simulink model "sys_dae"  (R2021a)
settings: Solver=VariableStepAuto  StartTime=0.0  StopTime=10.0  RelTol=1e-3
settings Model: Creator=Suman  LastModifiedBy=Suman

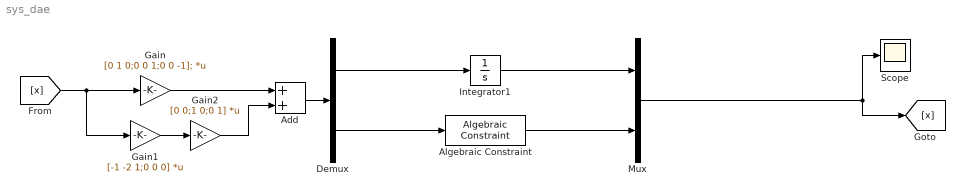
== system sys_dae ==
  Add : Sum
  Algebraic Constraint : AlgebraicConstraint
  Demux : Demux  Outputs=2
  Gain : Gain  Gain=[0 1 0;0 0 1;0 0 -1];  Multiplication=Matrix(K*u) (u vector)
  Gain1 : Gain  Gain=[-1 -2 1;0 0 0]  Multiplication=Matrix(K*u) (u vector)
  Gain2 : Gain  Gain=[0 0;1 0;0 1]  Multiplication=Matrix(K*u) (u vector)
  Integrator1 : Integrator  InitialCondition=[2;3]
  Mux : Mux  Inputs=2
  Scope : Scope
  wires:
  [x] -> Gain1/1, Gain/1
  Mux/1 -> Scope/1, [x]
  Demux/1 -> Integrator1/1
  Integrator1/1 -> Mux/1
  Demux/2 -> Algebraic Constraint/1
  Algebraic Constraint/1 -> Mux/2
  Add/1 -> Demux/1
  Gain/1 -> Add/1
  Gain1/1 -> Gain2/1
  Gain2/1 -> Add/2
